simulink model "Single_phase_PLL_System"  (R2025a)
settings: Solver=VariableStepAuto  StartTime=0.0  StopTime=10.0  RelTol=1e-3
InitFcn:
  | Wc = 1;
  | 
  | T = 0.001;
  | 
  | Kp = 0.8;
  | Ki = 1.2;
undefined symbols (not defined in the file): dspblkCoreblockFVToolHelper, gcbh
libraries: simulink x1
settings Model: Creator=星必尘Sguan  LastModifiedBy=星必尘Sguan
settings SFSimCC: SimCustomHeaderCode="#include \"PLL_SingleLoop.h\""  SimCustomInitializer=PLL_SingleInit();  SimUserSources=PLL_SingleLoop.c

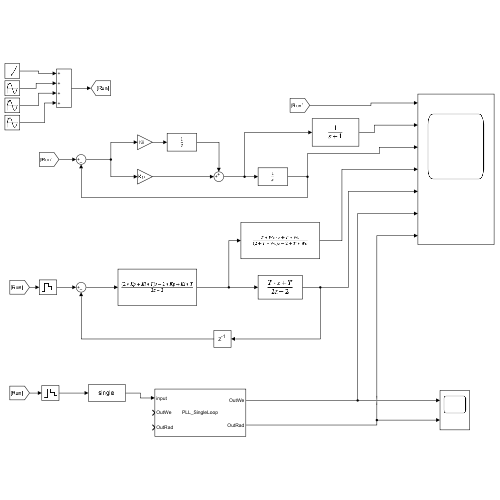
[thumbnail: Simulink's stored preview of the top-level diagram]
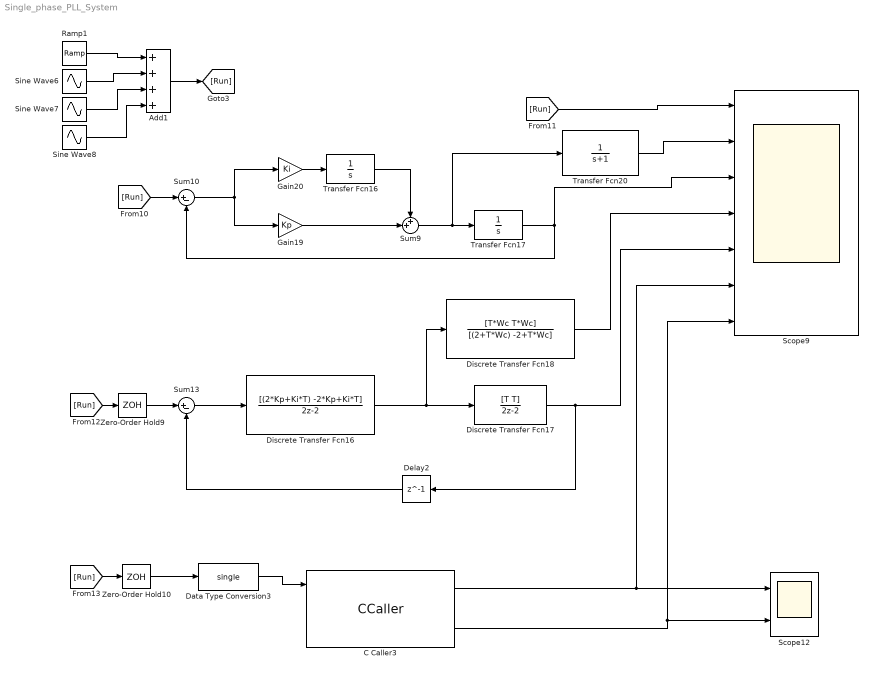
== system Single_phase_PLL_System ==
  Add1 : Sum  Inputs=++++
  C Caller3 : CCaller  FunctionName=PLL_SingleLoop  PortSpecificationStruct="%)30     .    F 4   8    (     @         %    \"     ,    !     0         %  0 \"0    $    _    07)G3F%M90  4&]R=$YA;64 4V-O<&4     26YD97@     5'EP90      4VEZ90      27-';&]B86P   X    X    !@    @    $          4    (     0    4    !         !     %    :6YP=70    .    .     8    (    !          %    \"     $    %     0         0    !0   &EN<'5T    #@   #@    &    \"     0         !0    @    !    !0    $         $     4   !);G!U=     X    X    !@    @    &          4    (     0    $    !          D    (               .    .     8    (    !          %    \"     $    &     0         0    !@   '-I;F=L90  #@   #     &    \"     0         !0    @    !     0    $         $  ! #$    .    ,     8    (    \"0(        %    \"     $    !     0         \"  $       X    X    !@    @    $          4    (     0    4    !         !     %    3W5T5V4    .    .     8    (    !          %    \"     $    %     0         0    !0   $]U=%=E    #@   $     &    \"     0         !0    @    !    \"P    $         $     L   !);G!U=$]U='!U=       #@   #@    &    \"     8         !0    @    !     0    $         \"0    @           #P/PX    X    !@    @    $          4    (     0    8    !         !     &    <VEN9VQE   .    ,     8    (    !          %    \"     $    \"     0         0  ( +3$   X    P    !@    @    ) @        4    (     0    $    !          (  0      #@   #@    &    \"     0         !0    @    !    !@    $         $     8   !/=712860   X    X    !@    @    $          4    (     0    8    !         !     &    3W5T4F%D   .    0     8    (    !          %    \"     $    +     0         0    \"P   $EN<'5T3W5T<'5T       .    .     8    (    !@         %    \"     $    !     0         )    \"             ! #@   #@    &    \"     0         !0    @    !    !@    $         $     8   !S:6YG;&4   X    P    !@    @    $          4    (     0    (    !         !   @ M,0  #@   #     &    \"     D\"        !0    @    !     0    $          @ !"
  Data Type Conversion3 : DataTypeConversion  OutDataTypeStr=single  SaturateOnIntegerOverflow=off  RndMeth=Floor
  Delay2 : Delay  DelayLength=1
  Discrete Transfer Fcn16 : DiscreteTransferFcn  LoadFcn=dspblkCoreblockFVToolHelper(gcbh,'load');  Numerator=[(2*Kp+Ki*T) -2*Kp+Ki*T]  Denominator=[2 -2]
      settings: CopyFcn=dspblkCoreblockFVToolHelper(gcbh,'copy');  DeleteFcn=dspblkCoreblockFVToolHelper(gcbh,'close');  ModelCloseFcn=dspblkCoreblockFVToolHelper(gcbh,'close');  PreSaveFcn=dspblkCoreblockFVToolHelper(gcbh,'presave');  PostSaveFcn=dspblkCoreblockFVToolHelper(gcbh,'postsave');  CloseFcn=dspblkCoreblockFVToolHelper(gcbh,'close');
  Discrete Transfer Fcn17 : DiscreteTransferFcn  LoadFcn=dspblkCoreblockFVToolHelper(gcbh,'load');  Numerator=[T T]  Denominator=[2 -2]
      settings: CopyFcn=dspblkCoreblockFVToolHelper(gcbh,'copy');  DeleteFcn=dspblkCoreblockFVToolHelper(gcbh,'close');  ModelCloseFcn=dspblkCoreblockFVToolHelper(gcbh,'close');  PreSaveFcn=dspblkCoreblockFVToolHelper(gcbh,'presave');  PostSaveFcn=dspblkCoreblockFVToolHelper(gcbh,'postsave');  CloseFcn=dspblkCoreblockFVToolHelper(gcbh,'close');
  Discrete Transfer Fcn18 : DiscreteTransferFcn  LoadFcn=dspblkCoreblockFVToolHelper(gcbh,'load');  Numerator=[T*Wc T*Wc]  Denominator=[(2+T*Wc) -2+T*Wc]
      settings: CopyFcn=dspblkCoreblockFVToolHelper(gcbh,'copy');  DeleteFcn=dspblkCoreblockFVToolHelper(gcbh,'close');  ModelCloseFcn=dspblkCoreblockFVToolHelper(gcbh,'close');  PreSaveFcn=dspblkCoreblockFVToolHelper(gcbh,'presave');  PostSaveFcn=dspblkCoreblockFVToolHelper(gcbh,'postsave');  CloseFcn=dspblkCoreblockFVToolHelper(gcbh,'close');
  Gain19 : Gain  Gain=Kp
  Gain20 : Gain  Gain=Ki
  Ramp1 : simulink/Sources/Ramp  slope=1  start=0  InitialOutput=0
  Scope12 : Scope  NumInputPorts=2
      settings: ActiveDisplayYMinimum=-1.251925468444824  ActiveDisplayYMaximum=11.267329216003418  DataLoggingVariableName=ScopeData13
  Scope9 : Scope  NumInputPorts=7
      settings: ActiveDisplayYMinimum=-1.8025038091260754  ActiveDisplayYMaximum=11.854858515541672  DataLoggingVariableName=ScopeData10
  Sine Wave6 : Sin  Amplitude=0.3  Frequency=80  SampleTime=0
  Sine Wave7 : Sin  Amplitude=0.2  Frequency=300  SampleTime=0
  Sine Wave8 : Sin  Amplitude=0.003  Frequency=1000  SampleTime=0
  Sum10 : Sum  Inputs=|+-
  Sum13 : Sum  Inputs=|+-
  Sum9 : Sum  Inputs=++|
  Transfer Fcn16 : TransferFcn  Denominator=[1 0]
  Transfer Fcn17 : TransferFcn  Denominator=[1 0]
  Transfer Fcn20 : TransferFcn  Denominator=[1 1]
  Zero-Order Hold10 : ZeroOrderHold  SampleTime=0.001
  Zero-Order Hold9 : ZeroOrderHold  SampleTime=0.001
  wires:
  Transfer Fcn17/1 -> Sum10/2, Scope9/3
  Sum10/1 -> Gain19/1, Gain20/1
  [Run] -> Scope9/1
  [Run] -> Sum10/1
  Zero-Order Hold10/1 -> Data Type Conversion3/1
  Zero-Order Hold9/1 -> Sum13/1
  Transfer Fcn16/1 -> Sum9/1
  Sum9/1 -> Transfer Fcn20/1, Transfer Fcn17/1
  Gain19/1 -> Sum9/2
  [Run] -> Zero-Order Hold9/1
  Discrete Transfer Fcn17/1 -> Scope9/5, Delay2/1
  Transfer Fcn20/1 -> Scope9/2
  Discrete Transfer Fcn18/1 -> Scope9/4
  Gain20/1 -> Transfer Fcn16/1
  C Caller3/1 -> Scope12/1, Scope9/6
  [Run] -> Zero-Order Hold10/1
  Discrete Transfer Fcn16/1 -> Discrete Transfer Fcn18/1, Discrete Transfer Fcn17/1
  Data Type Conversion3/1 -> C Caller3/1
  Sum13/1 -> Discrete Transfer Fcn16/1
  C Caller3/2 -> Scope12/2, Scope9/7
  Delay2/1 -> Sum13/2
  Sine Wave7/1 -> Add1/3
  Sine Wave6/1 -> Add1/2
  Add1/1 -> [Run]
  Sine Wave8/1 -> Add1/4
  Ramp1/1 -> Add1/1
